simulink library "intertravamento"  (R2015a)
settings: Solver=ode45  SolverMode=SingleTasking  StartTime=0.0  StopTime=10.0  RelTol=1e-3
PostLoadFcn:
  | setsysloc_simulink(bdroot)
undefined symbols (not defined in the file or in its folder): docblock, getdatatypespecs, NumBits1, NumBits2, sfunxy, sigbuilder_block, slcm, SlDemoSign, Slope1, Slope2
libraries: simulink x46, sl_helperblocks x2, eml_lib x1
(part 6 of 6)

== system intertravamento/Model-Wide Utilities/Block Support Table ==
  EmptySubsystem : Subsystem

== system intertravamento/Model-Wide Utilities/DocBlock ==
  EmptySubsystem : Subsystem

== system intertravamento/Model-Wide Utilities/Model Info ==
  EmptySubsystem : Subsystem

== system intertravamento/Model-Wide Utilities/Timed-Based Linearization ==
  Clock : Clock
      settings: DisableCoverage=on
  Constant : Constant  DisableCoverage=on  Value=LinearizationTime
  Sum : Sum  DisableCoverage=on  Inputs=-+  SaturateOnIntegerOverflow=on  InputSameDT=on  OutDataTypeStr=Inherit: Same as first input
  Triggered Linearization : Subsystem  DisableCoverage=on  TreatAsAtomicUnit=on
  wires:
  Clock/1 -> Sum/2
  Constant/1 -> Sum/1
  Sum/1 -> Triggered Linearization/Trigger

== system intertravamento/Model-Wide Utilities/Trigger-Based Linearization ==
  Trigger : TriggerPort
  MATLAB S-Function : M-S-Function  DisableCoverage=on  FunctionName=sfunlin  Parameters=name_,SampleTime

== system intertravamento/Ports & Subsystems/Atomic Subsystem ==
  In1 : Inport
  Out1 : Outport
  wires:
  In1/1 -> Out1/1

== system intertravamento/Ports & Subsystems/CodeReuseSubsystem ==
  In1 : Inport
  Out1 : Outport
  wires:
  In1/1 -> Out1/1

== system intertravamento/Ports & Subsystems/Configurable Subsystem ==

== system intertravamento/Ports & Subsystems/Enabled Subsystem ==
  In1 : Inport
  Enable : EnablePort
  Out1 : Outport
  wires:
  In1/1 -> Out1/1

== system intertravamento/Ports & Subsystems/Enabled and Triggered Subsystem ==
  In1 : Inport
  Enable : EnablePort
  Trigger : TriggerPort
  Out1 : Outport
  wires:
  In1/1 -> Out1/1

== system intertravamento/Ports & Subsystems/For Each Subsystem ==
  In1 : Inport  Partition=on  PartitionDimension=1  PartitionWidth=1
  For Each : ForEach  DisableCoverage=on  IndexMode=One-based
  Out1 : Outport  ConcatenationDimension=1
  wires:
  In1/1 -> Out1/1

== system intertravamento/Ports & Subsystems/For Iterator Subsystem ==
  In1 : Inport
  For Iterator : ForIterator
  Out1 : Outport
  wires:
  In1/1 -> Out1/1

== system intertravamento/Ports & Subsystems/Function-Call Subsystem ==
  In1 : Inport
  function : TriggerPort  TriggerType=function-call
  Out1 : Outport
  wires:
  In1/1 -> Out1/1

== system intertravamento/Ports & Subsystems/If Action Subsystem ==
  In1 : Inport
  Action Port : ActionPort  ActionType=then
  Out1 : Outport
  wires:
  In1/1 -> Out1/1

== system intertravamento/Ports & Subsystems/Resettable Subsystem ==
  In1 : Inport
  Reset : ResetPort  DisableCoverage=on
  Out1 : Outport
  wires:
  In1/1 -> Out1/1

== system intertravamento/Ports & Subsystems/Subsystem ==
  In1 : Inport
  Out1 : Outport
  wires:
  In1/1 -> Out1/1

== system intertravamento/Ports & Subsystems/Subsystem Examples ==
  Gain : Gain  SaturateOnIntegerOverflow=on  OutDataTypeStr=Inherit: Same as input  ParamDataTypeStr=Inherit: Same as input

== system intertravamento/Ports & Subsystems/Switch Case Action Subsystem ==
  In1 : Inport
  Action Port : ActionPort  ActionType=case
  Out1 : Outport
  wires:
  In1/1 -> Out1/1

== system intertravamento/Ports & Subsystems/Triggered Subsystem ==
  In1 : Inport
  Trigger : TriggerPort
  Out1 : Outport
  wires:
  In1/1 -> Out1/1

== system intertravamento/Ports & Subsystems/Variant Subsystem ==
  note: 1) Add Subsystem or Model blocks as valid variant choices.
      | 2) You cannot connect blocks at this level. At simulation, connectivity is automatically
      | determined, based on the active variant and port name matching.
  In1 : Inport
  Out1 : Outport

== system intertravamento/Ports & Subsystems/While Iterator Subsystem ==
  In1 : Inport
  IC : Inport  Port=2
  While Iterator : WhileIterator
  Out1 : Outport
  wires:
  In1/1 -> Out1/1
  IC/1 -> While Iterator/2

== system intertravamento/Signal Attributes/Data Type Conversion Inherited ==
  DTS reference : Inport
  u : Inport  Port=2
  Conversion : DataTypeConversion  LockScale=on
  Data Type Duplicate : DataTypeDuplicate  DisableCoverage=on
  y : Outport
  wires:
  u/1 -> Conversion/1
  DTS reference/1 -> Data Type Duplicate/1
  Conversion/1 -> y/1, Data Type Duplicate/2

== system intertravamento/Signal Attributes/Data Type Propagation Examples ==
  Gain : Gain  SaturateOnIntegerOverflow=on  OutDataTypeStr=Inherit: Same as input  ParamDataTypeStr=Inherit: Same as input

== system intertravamento/Signal Attributes/Data Type Scaling Strip ==
  note: Force Scaling to be nominal,
      | slope == 1.0
      | bias == 0.0
  note: Gateway Out set to "auto"
      | which is similar to
      | "Inherit via back propagation"
  u : Inport
  FixPt Data Type Propagation : simulink/Signal Attributes/Data Type Propagation  PropDataType=fixdt(1, 16)  IfRefDouble=double  IfRefSingle=single  IsSigned=IsSigned1  NumBitsBase=NumBits1  NumBitsMult=1  NumBitsAdd=0  NumBitsAllowFinal=[8,16,32,128]  PropScalingMode=Specify via dialog  PropScaling=1  ValuesUsedBestPrec=[5 -7]  SlopeBase=Slope1  SlopeMult=0  SlopeAdd=1  BiasBase=Bias1  BiasMult=1  BiasAdd=0
  FixPt Gateway Out : DataTypeConversion  ConvertRealWorld=Stored Integer (SI)
  y : Outport
  wires:
  u/1 -> FixPt Data Type Propagation/1, FixPt Data Type Propagation/2, FixPt Gateway Out/1
  FixPt Gateway Out/1 -> FixPt Data Type Propagation/3, y/1

== system intertravamento/Signal Routing/Environment Controller ==
  Sim : Inport
  Coder : Inport  Port=2
  Environment Switch : Switch  DisableCoverage=on  Criteria=u2 ~= 0  ZeroCross=off  InputSameDT=on
  Numerical Unity : SignalConversion
  Switch Control : Constant  DisableCoverage=on  Value=switch_mode  OutDataTypeStr=boolean
  Out : Outport
  wires:
  Sim/1 -> Environment Switch/1
  Switch Control/1 -> Environment Switch/2
  Environment Switch/1 -> Numerical Unity/1
  Coder/1 -> Environment Switch/3
  Numerical Unity/1 -> Out/1

== system intertravamento/Sinks/XY Graph ==
  x : Inport
  y : Inport  Port=2
  Data Type Conversion : DataTypeConversion  DisableCoverage=on  OutDataTypeStr=double
  Data Type Conversion1 : DataTypeConversion  DisableCoverage=on  OutDataTypeStr=double
  Mux : Mux  Inputs=2
  sfunxy : S-Function  DisableCoverage=on  FunctionName=sfunxy  Parameters=[xmin xmax ymin ymax], st
  wires:
  Mux/1 -> sfunxy/1
  x/1 -> Data Type Conversion/1
  y/1 -> Data Type Conversion1/1
  Data Type Conversion/1 -> Mux/1
  Data Type Conversion1/1 -> Mux/2

== system intertravamento/Sources/Band-Limited White Noise ==
  Output : Gain  Gain=[sqrt(Cov)]/[sqrt(Ts)]  SaturateOnIntegerOverflow=on  OutDataTypeStr=Inherit: Same as input  ParamDataTypeStr=Inherit: Same as input
  White Noise : RandomNumber  DisableCoverage=on  Seed=seed  SampleTime=Ts
  y : Outport
  wires:
  White Noise/1 -> Output/1
  Output/1 -> y/1

== system intertravamento/Sources/Chirp Signal ==
  note: freqSlope = deltaFreq/targetTime;
      | instantaneousFreq(t) = freqSlope*t + initialFreq;
      | intantaneousPhase(t) = integral(instFreq) = ...
      |       0.5*freqSlope*t^2 + initialFreq*t;
      | outputSignal(t) = sin(instantaneousPhase(t));
  Clock1 : Clock
      settings: DisableCoverage=on
  Gain : Gain  DisableCoverage=on  Gain=0.5  OutDataTypeStr=Inherit: Same as input  ParamDataTypeStr=Inherit: Same as input
  Output : Trigonometry
  Product : Product  DisableCoverage=on  Inputs=*/  SaturateOnIntegerOverflow=on  InputSameDT=on  OutDataTypeStr=Inherit: Same as first input
  Product1 : Product  DisableCoverage=on  SaturateOnIntegerOverflow=on  InputSameDT=on  OutDataTypeStr=Inherit: Same as first input
  Product2 : Product  DisableCoverage=on  SaturateOnIntegerOverflow=on  InputSameDT=on  OutDataTypeStr=Inherit: Same as first input
  Sum : Sum  DisableCoverage=on  Inputs=|++  SaturateOnIntegerOverflow=on  InputSameDT=on  OutDataTypeStr=Inherit: Same as first input
  deltaFreq : Constant  DisableCoverage=on  Value=2*pi*(f2-f1)
  initialFreq : Constant  DisableCoverage=on  Value=2*pi*f1
  targetTime : Constant  DisableCoverage=on  Value=T
  y : Outport
  wires:
  deltaFreq/1 -> Product/1
  targetTime/1 -> Product/2
  Product/1 -> Gain/1
  Clock1/1 -> Product1/1, Product2/1
  Gain/1 -> Product1/2
  Product1/1 -> Sum/1
  initialFreq/1 -> Sum/2
  Sum/1 -> Product2/2
  Product2/1 -> Output/1
  Output/1 -> y/1

== system intertravamento/Sources/Counter Free-Running ==
  FixPt Data Type Propagation : simulink/Signal Attributes/Data Type Propagation  PropDataTypeMode=Specify via dialog  PropDataType=uint(NumBits)  IfRefDouble=double  IfRefSingle=single  IsSigned=IsSigned1 or IsSigned2  NumBitsBase=max([NumBits1 NumBits2])  NumBitsMult=1  NumBitsAdd=0  NumBitsAllowFinal=1:128  PropScalingMode=Specify via dialog  PropScaling=1  ValuesUsedBestPrec=[5 -7]  SlopeBase=min([Slope1 Slope2])  SlopeMult=1  SlopeAdd=0  BiasBase=Bias1  BiasMult=1  BiasAdd=0
  Force to be scalar : SignalSpecification  DisableCoverage=on  Dimensions=1
  Increment Real World : simulink/Additional Math & Discrete/Additional Math: Increment - Decrement/Increment Real World  DisableCoverage=on
  Output : UnitDelay  InitialCondition=0.0  SampleTime=tsamp
  Wrap To Zero : simulink/Discontinuities/Wrap To Zero  DisableCoverage=on  Threshold=(2^(NumBits))-1
  y : Outport
  wires:
  Force to be scalar/1 -> Increment Real World/1
  Wrap To Zero/1 -> Output/1, FixPt Data Type Propagation/1, FixPt Data Type Propagation/3, FixPt Data Type Propagation/2
  Increment Real World/1 -> Wrap To Zero/1
  Output/1 -> Force to be scalar/1, y/1

== system intertravamento/Sources/Counter Limited ==
  Data Type Propagation : simulink/Signal Attributes/Data Type Propagation  PropDataTypeMode=Specify via dialog  PropDataType=uint(nbits)  IfRefDouble=double  IfRefSingle=single  IsSigned=IsSigned1 or IsSigned2  NumBitsBase=max([NumBits1 NumBits2])  NumBitsMult=1  NumBitsAdd=0  NumBitsAllowFinal=1:128  PropScalingMode=Specify via dialog  PropScaling=1  ValuesUsedBestPrec=[5 -7]  SlopeBase=min([Slope1 Slope2])  SlopeMult=1  SlopeAdd=0  BiasBase=Bias1  BiasMult=1  BiasAdd=0
  Force to be scalar : SignalSpecification  DisableCoverage=on  Dimensions=1
  Increment Real World : simulink/Additional Math & Discrete/Additional Math: Increment - Decrement/Increment Real World  DisableCoverage=on
  Output : UnitDelay  InitialCondition=0.0  SampleTime=tsamp
  Wrap To Zero : simulink/Discontinuities/Wrap To Zero  DisableCoverage=on  Threshold=uplimit
  y : Outport
  wires:
  Force to be scalar/1 -> Increment Real World/1
  Increment Real World/1 -> Wrap To Zero/1
  Output/1 -> Force to be scalar/1, y/1
  Wrap To Zero/1 -> Data Type Propagation/3, Data Type Propagation/2, Data Type Propagation/1, Output/1

== system intertravamento/Sources/Enumerated Constant ==
  Constant : Constant  DialogController=Simulink.DDGSource  Value=SlDemoSign.Positive  OutDataTypeStr=Enum: SlDemoSign  LockScale=on
  Out : Outport
  wires:
  Constant/1 -> Out/1

== system intertravamento/Sources/Ramp ==
  Clock : Clock
      settings: DisableCoverage=on
  Constant : Constant  DisableCoverage=on  Value=start  OutDataTypeStr=Inherit: Inherit via back propagation
  Constant1 : Constant  DisableCoverage=on  Value=X0  OutDataTypeStr=Inherit: Inherit via back propagation
  Output : Sum  Inputs=|++  SaturateOnIntegerOverflow=on  InputSameDT=on  OutDataTypeStr=Inherit: Same as first input
  Product : Product  DisableCoverage=on  SaturateOnIntegerOverflow=on  InputSameDT=on  OutDataTypeStr=Inherit: Same as first input
  Step : Step  DisableCoverage=on  Time=start  After=slope  SampleTime=0
  Sum : Sum  DisableCoverage=on  Inputs=|+-  SaturateOnIntegerOverflow=on  InputSameDT=on  OutDataTypeStr=Inherit: Same as first input
  Out1 : Outport
  wires:
  Step/1 -> Product/1
  Product/1 -> Output/1
  Constant1/1 -> Output/2
  Output/1 -> Out1/1
  Sum/1 -> Product/2
  Constant/1 -> Sum/2
  Clock/1 -> Sum/1

== system intertravamento/Sources/Repeating Sequence ==
  Clock : Clock
      settings: DisableCoverage=on
  Constant : Constant  DisableCoverage=on  Value=period
  Look-Up Table1 : Lookup_n-D  DisableCoverage=on  NumberOfTableDimensions=1  BreakpointsForDimension1=rep_seq_t - min(rep_seq_t)  BreakpointsForDimension3=[5, 7]  Table=rep_seq_y  InternalRulePriority=Speed  SaturateOnIntegerOverflow=on  InputSameDT=on
  Math Function : Math  DisableCoverage=on  Operator=rem  SaturateOnIntegerOverflow=on
  Output : SignalConversion
  Sum : Sum  DisableCoverage=on  Inputs=+-  SaturateOnIntegerOverflow=on  InputSameDT=on  OutDataTypeStr=Inherit: Same as first input
  startTime : S-Function  DisableCoverage=on  FunctionName=sfun_tstart
  Out1 : Outport
  wires:
  Math Function/1 -> Look-Up Table1/1
  Sum/1 -> Math Function/1
  Clock/1 -> Sum/1
  startTime/1 -> Sum/2
  Look-Up Table1/1 -> Output/1
  Output/1 -> Out1/1
  Constant/1 -> Math Function/2

== system intertravamento/Sources/Repeating Sequence Interpolated ==
  Data Type Propagation : simulink/Signal Attributes/Data Type Propagation  PropDataType=fixdt(1, 16)  IfRefDouble=double  IfRefSingle=single  IsSigned=IsSigned2  NumBitsBase=NumBits2  NumBitsMult=1  NumBitsAdd=0  NumBitsAllowFinal=1:128  PropScaling=2^-10  ValuesUsedBestPrec=[5 -7]  SlopeBase=Slope2  SlopeMult=1  SlopeAdd=0  BiasBase=Bias2  BiasMult=1  BiasAdd=0
  Data Type Conversion : DataTypeConversion  DisableCoverage=on
  Force to be scalar : SignalSpecification  DisableCoverage=on  Dimensions=1
  LimitedCounter : simulink/Sources/Counter Limited  uplimit=nn  tsamp=tsamp
  Lookup : Lookup_n-D  DisableCoverage=on  NumberOfTableDimensions=1  BreakpointsForDimension1=TimeValues  BreakpointsForDimension3=[5, 7]  Table=OutValues  ExtrapMethod=Clip  OutMin=OutMin  OutMax=OutMax  OutDataTypeStr=OutDataTypeStr  InputSameDT=on
  Output : SignalConversion
  Sample Time Math : SampleTimeMath  DisableCoverage=on  TsampMathOp=*  TsampMathImp=Offline Scaling Adjustment
  y : Outport  OutMin=OutMin  OutMax=OutMax
  wires:
  Output/1 -> y/1
  Lookup/1 -> Output/1, Data Type Propagation/1
  Force to be scalar/1 -> Data Type Conversion/1, Data Type Propagation/2
  LimitedCounter/1 -> Force to be scalar/1
  Sample Time Math/1 -> Lookup/1
  Data Type Conversion/1 -> Sample Time Math/1, Data Type Propagation/3

== system intertravamento/Sources/Repeating Sequence Stair ==
  Force to be scalar : SignalSpecification  DisableCoverage=on  Dimensions=1
  LimitedCounter : simulink/Sources/Counter Limited  uplimit=nn  tsamp=tsamp
  Out : SignalConversion
  Output : MultiPortSwitch  DisableCoverage=on  DataPortOrder=Zero-based contiguous  Inputs=1  zeroidx=on  OutMin=OutMin  OutMax=OutMax  SampleTime=tsamp
  Vector : Constant  DisableCoverage=on  Value=OutValues  OutMin=OutMin  OutMax=OutMax  OutDataTypeStr=OutDataTypeStr
  y : Outport  OutMin=OutMin  OutMax=OutMax
  wires:
  Force to be scalar/1 -> Output/1
  Vector/1 -> Output/2
  LimitedCounter/1 -> Force to be scalar/1
  Output/1 -> Out/1
  Out/1 -> y/1

== system intertravamento/Sources/Signal Builder ==
  Demux : Demux  Tag=STV Demux  Outputs=1
  FromWs : FromWorkspace  Tag=STV FromWs  VariableName=tuvar  SampleTime=0
      SigBuilderData=|
      | common.afterFinalStr = 'Extrapolate'
      | common.sampleTime = 0
      | dataSet.timeRange = [0 10]
      | dataSet.name = 'Group 1'
      | sbobj.Groups.Name = 'Group 1'
      | sbobj.Groups.Signals.Name = 'Signal 1'
      | sbobj.Groups.Signals.XData = [0 4 4 6 6 10]
      | sbobj.Groups.Signals.YData = [0 0 1 1 0 0]
  Signal 1 : Outport  Tag=STV Outport
  wires:
  FromWs/1 -> Demux/1
  Demux/1 -> Signal 1/1

== system intertravamento/User-Defined Functions/S-Function Examples ==
  Gain : Gain  SaturateOnIntegerOverflow=on  OutDataTypeStr=Inherit: Same as input  ParamDataTypeStr=Inherit: Same as input

== system intertravamento/User-Defined Functions/Simulink Function ==
  f : TriggerPort  TriggerType=function-call  IsSimulinkFunction=on  FunctionName=f
  u : ArgIn  DisableCoverage=on  ArgumentName=u
  y : ArgOut  DisableCoverage=on  ArgumentName=y
  wires:
  u/1 -> y/1

== system intertravamento/Additional Math & Discrete/Additional Discrete/Fixed-Point State-Space ==
  note: U(k)
  note: U(k)
  note: Y(k)
  u : Inport
  Data Type Duplicate : DataTypeDuplicate  DisableCoverage=on  NumInputPorts=3
  Data Type Duplicate1 : DataTypeDuplicate  DisableCoverage=on  NumInputPorts=3
  DataTypeProp : simulink/Signal Attributes/Data Type Propagation  PropDataType=fixdt(1, 16)  IfRefDouble=double  IfRefSingle=single  IsSigned=IsSigned1 or IsSigned2  NumBitsBase=NumBits1  NumBitsMult=1  NumBitsAdd=0  NumBitsAllowFinal=1:128  PropScaling=2^-10  ValuesUsedBestPrec=[5 -7]  SlopeBase=PosRange2  SlopeMult=1  SlopeAdd=0  BiasBase=Bias2  BiasMult=1  BiasAdd=0
  DataTypeProp1 : simulink/Signal Attributes/Data Type Propagation  PropDataType=fixdt(1, 16)  IfRefDouble=double  IfRefSingle=single  IsSigned=IsSigned1 or IsSigned2  NumBitsBase=NumBits1  NumBitsMult=1  NumBitsAdd=0  NumBitsAllowFinal=1:128  PropScaling=2^-10  ValuesUsedBestPrec=[5 -7]  SlopeBase=PosRange2  SlopeMult=1  SlopeAdd=0  BiasBase=Bias2  BiasMult=1  BiasAdd=0
  Delay State X : UnitDelay  Description=Store in Global RAM  DisableCoverage=on  InitialCondition=X0  SampleTime=-1
      settings: AttributesFormatString=%<Description>
  Direct Link Matrix D : Gain  Description=Multiply in CPU  DisableCoverage=on  Gain=D  Multiplication=Matrix(K*u) (u vector)  OutDataTypeStr=Inherit: Inherit via back propagation
      settings: AttributesFormatString=%<Description>
  Downcast Next State X : DataTypeConversion  Description=|  DisableCoverage=on
      | Reduce from CPU Size
      |  to Global RAM Size
      settings: AttributesFormatString=%<Description>
  Downcast Output Y : DataTypeConversion  Description=|
      | Reduce from CPU Size
      |  to Global RAM Size
      settings: AttributesFormatString=%<Description>
  Input Matrix B : Gain  Description=Multiply in CPU  DisableCoverage=on  Gain=B  Multiplication=Matrix(K*u) (u vector)  OutDataTypeStr=Inherit: Inherit via back propagation
      settings: AttributesFormatString=%<Description>
  Output Matrix C : Gain  Description=Multiply in CPU  DisableCoverage=on  Gain=C  Multiplication=Matrix(K*u) (u vector)  OutDataTypeStr=Inherit: Inherit via back propagation
      settings: AttributesFormatString=%<Description>
  State Matrix A : Gain  Description=Multiply in CPU  DisableCoverage=on  Gain=A  Multiplication=Matrix(K*u) (u vector)  OutDataTypeStr=Inherit: Inherit via back propagation
      settings: AttributesFormatString=%<Description>
  Sum Output Equation : Sum  Description=Add in CPU  DisableCoverage=on  OutDataTypeStr=slDataTypeAndScale(('InternalDataType'),('OutputEqScaling'))
      settings: AttributesFormatString=%<Description>
  Sum State Equation : Sum  Description=Add in CPU  DisableCoverage=on  OutDataTypeStr=slDataTypeAndScale(('InternalDataType'),('StateEqScaling'))
      settings: AttributesFormatString=%<Description>
  y : Outport  InitialOutput=0
  wires:
  Direct Link Matrix D/1 -> Data Type Duplicate1/3, Sum Output Equation/1  "DU(k)"
  Output Matrix C/1 -> Data Type Duplicate1/2, Sum Output Equation/2  "CX(k)"
  Sum Output Equation/1 -> DataTypeProp/2, Data Type Duplicate1/1, Downcast Output Y/1  "CX(k)+DU(k)"
  Downcast Output Y/1 -> DataTypeProp/3, y/1
  Delay State X/1 -> Output Matrix C/1, State Matrix A/1  "X(k)"
  Downcast Next State X/1 -> DataTypeProp1/3, Delay State X/1  "X(k+1)"
  Sum State Equation/1 -> DataTypeProp1/2, Data Type Duplicate/1, Downcast Next State X/1  "AX(k)+BU(k)"
  Input Matrix B/1 -> Data Type Duplicate/3, Sum State Equation/1  "BU(k)"
  u/1 -> DataTypeProp1/1, DataTypeProp/1, Direct Link Matrix D/1, Input Matrix B/1
  State Matrix A/1 -> Data Type Duplicate/2, Sum State Equation/2  "AX(k)"

== system intertravamento/Additional Math & Discrete/Additional Discrete/Transfer Fcn Direct Form II ==
  u : Inport
  DataTypeProp : simulink/Signal Attributes/Data Type Propagation  PropDataType=fixdt(1, 16)  IfRefDouble=double  IfRefSingle=single  IsSigned=IsSigned1 or IsSigned2  NumBitsBase=max([NumBits1 NumBits2])  NumBitsMult=1  NumBitsAdd=0  NumBitsAllowFinal=1:128  PropScaling=2^-10  ValuesUsedBestPrec=[5 -7]  SlopeBase=min([Slope1 Slope2])  SlopeMult=OutputSlopeMult  SlopeAdd=0  BiasBase=Bias1  BiasMult=0  BiasAdd=0
  DataTypeProp1 : simulink/Signal Attributes/Data Type Propagation  PropDataType=fixdt(1, 16)  IfRefDouble=double  IfRefSingle=single  IsSigned=IsSigned1 or IsSigned2  NumBitsBase=max([NumBits1 NumBits2])  NumBitsMult=1  NumBitsAdd=0  NumBitsAllowFinal=1:128  PropScaling=2^-10  ValuesUsedBestPrec=[5 -7]  SlopeBase=min([Slope1 Slope2])  SlopeMult=OutputSlopeMult2  SlopeAdd=0  BiasBase=Bias1  BiasMult=0  BiasAdd=0
  DenCoef : Gain  DisableCoverage=on  Gain=DenCoefVec  Multiplication=Matrix(K*u) (u vector)
      settings: AttributesFormatString=|
      | Data Type and Scaling Inherited
      | with goal of NO Quantization Noise
      | Possible Overflow or Saturation
  Downcast : DataTypeConversion  Description=|  LockScale=on
      | Reduce from CPU Size
      |  to Global RAM Size
      settings: AttributesFormatString=%<Description>
  Downcast1 : DataTypeConversion  Description=|  DisableCoverage=on  LockScale=on
      | Reduce from CPU Size
      |  to Global RAM Size
      settings: AttributesFormatString=%<Description>
  Mux : Mux  Inputs=2
  NumCoef : Gain  DisableCoverage=on  Gain=NumCoefVec  Multiplication=Matrix(K*u) (u vector)
      settings: AttributesFormatString=|
      | Data Type and Scaling Inherited
      | with goal of NO Quantization Noise
      | Possible Overflow or Saturation
  Sum : Sum  Tag=S16 2^-10  DisableCoverage=on  Inputs=+-  LockScale=on
      settings: AttributesFormatString=|
      | Data Type and Scaling Inherited
      | with goal of NO Quantization Noise
      | Possible Overflow or Saturation
  Tapped Delay : simulink/Discrete/Tapped Delay  vinit=vinit  samptime=-1  NumDelays=-1  DelayOrder=Newest  includeCurrent=off
      settings: AttributesFormatString=|
      | Number of Taps
      | Inherited via Back Propagation
  y : Outport
  wires:
  Sum/1 -> Downcast1/1
  DenCoef/1 -> Sum/2
  u/1 -> DataTypeProp1/1, DataTypeProp1/2, DataTypeProp/2, DataTypeProp/1, Sum/1
  NumCoef/1 -> Downcast/1
  Tapped Delay/1 -> DenCoef/1, Mux/2
  Downcast1/1 -> DataTypeProp1/3, Mux/1, Tapped Delay/1
  Mux/1 -> NumCoef/1
  Downcast/1 -> y/1, DataTypeProp/3

== system intertravamento/Additional Math & Discrete/Additional Discrete/Transfer Fcn Direct Form II Time Varying ==
  u : Inport
  Num : Inport  Port=2
  Den No Lead : Inport  Port=3
  DataTypeProp : simulink/Signal Attributes/Data Type Propagation  PropDataType=fixdt(1, 16)  IfRefDouble=double  IfRefSingle=single  IsSigned=IsSigned1  NumBitsBase=NumBits1  NumBitsMult=1  NumBitsAdd=0  NumBitsAllowFinal=1:128  PropScaling=2^-10  ValuesUsedBestPrec=[5 -7]  SlopeBase=Slope1  SlopeMult=1  SlopeAdd=0  BiasBase=Bias1  BiasMult=1  BiasAdd=0
  DataTypeProp1 : simulink/Signal Attributes/Data Type Propagation  PropDataType=fixdt(1, 16)  IfRefDouble=double  IfRefSingle=single  IsSigned=IsSigned1  NumBitsBase=NumBits1  NumBitsMult=1  NumBitsAdd=0  NumBitsAllowFinal=1:128  PropScaling=2^-10  ValuesUsedBestPrec=[5 -7]  SlopeBase=Slope1  SlopeMult=2  SlopeAdd=0  BiasBase=Bias1  BiasMult=1  BiasAdd=0
  Dot1 : DotProduct  DisableCoverage=on  OutDataTypeStr=Inherit: Inherit via internal rule
      settings: AttributesFormatString=|
      | Data Type and Scaling Inherited
      | with goal of NO Quantization Noise
      | Possible Overflow or Saturation
  Dot2 : DotProduct  DisableCoverage=on  OutDataTypeStr=Inherit: Inherit via internal rule
      settings: AttributesFormatString=|
      | Data Type and Scaling Inherited
      | with goal of NO Quantization Noise
      | Possible Overflow or Saturation
  Downcast : DataTypeConversion  Description=|  LockScale=on
      | Reduce from CPU Size
      |  to Global RAM Size
      settings: AttributesFormatString=%<Description>
  Downcast1 : DataTypeConversion  Description=|  DisableCoverage=on  LockScale=on
      | Reduce from CPU Size
      |  to Global RAM Size
      settings: AttributesFormatString=%<Description>
  Mux : Mux  Inputs=2
  Sum : Sum  Tag=S16 2^-10  DisableCoverage=on  Inputs=+-  LockScale=on
      settings: AttributesFormatString=|
      | Data Type and Scaling Inherited
      | with goal of NO Quantization Noise
      | Possible Overflow or Saturation
  Tapped Delay : simulink/Discrete/Tapped Delay  vinit=vinit  samptime=-1  NumDelays=-1  DelayOrder=Newest  includeCurrent=off
      settings: AttributesFormatString=|
      | Number of Taps
      | Inherited via Back Propagation
  y : Outport
  wires:
  Den No Lead/1 -> Dot1/2
  Num/1 -> Dot2/2
  Downcast/1 -> DataTypeProp/3, y/1
  Mux/1 -> Dot2/1
  Downcast1/1 -> DataTypeProp1/3, Tapped Delay/1, Mux/1
  Tapped Delay/1 -> Dot1/1, Mux/2
  Dot2/1 -> Downcast/1
  u/1 -> Sum/1, DataTypeProp1/2, DataTypeProp1/1, DataTypeProp/2, DataTypeProp/1
  Dot1/1 -> Sum/2
  Sum/1 -> Downcast1/1

== system intertravamento/Additional Math & Discrete/Additional Discrete/Unit Delay Enabled ==
  note: Enable
  note: Xold
  u : Inport
  E : Inport  Port=2
  Enable : Switch  Criteria=u2 ~= 0  OutDataTypeStr=Inherit: Inherit via back propagation  ZeroCross=off
  FixPt Data Type Duplicate1 : DataTypeDuplicate  DisableCoverage=on  NumInputPorts=3
  FixPt Unit Delay1 : UnitDelay  InitialCondition=vinit  SampleTime=tsamp  HasFrameUpgradeWarning=off
  y : Outport
  wires:
  E/1 -> Enable/2
  u/1 -> FixPt Data Type Duplicate1/3, Enable/1
  Enable/1 -> FixPt Unit Delay1/1, FixPt Data Type Duplicate1/2  "Xnew"
  FixPt Unit Delay1/1 -> y/1, Enable/3, FixPt Data Type Duplicate1/1

== system intertravamento/Additional Math & Discrete/Additional Discrete/Unit Delay Enabled External IC ==
  note: Enable
  note: Initial Value
  u : Inport
  E : Inport  Port=2
  IC : Inport  Port=3
  Enable : Switch  Criteria=u2 ~= 0  OutDataTypeStr=Inherit: Inherit via back propagation  ZeroCross=off
  FixPt Data Type Duplicate1 : DataTypeDuplicate  DisableCoverage=on  NumInputPorts=4
  Unit Delay External IC : simulink/Additional Math & Discrete/Additional Discrete/Unit Delay External IC  tsamp=tsamp
  y : Outport
  wires:
  E/1 -> Enable/2
  IC/1 -> FixPt Data Type Duplicate1/3, Unit Delay External IC/2
  u/1 -> FixPt Data Type Duplicate1/4, Enable/1
  Enable/1 -> FixPt Data Type Duplicate1/2, Unit Delay External IC/1  "Xnew"
  Unit Delay External IC/1 -> y/1, Enable/3, FixPt Data Type Duplicate1/1

== system intertravamento/Additional Math & Discrete/Additional Discrete/Unit Delay Enabled Resettable ==
  note: Enable
  note: Reset
  u : Inport
  E : Inport  Port=2
  R : Inport  Port=3
  Enable : Switch  Criteria=u2 ~= 0  OutDataTypeStr=Inherit: Inherit via back propagation  ZeroCross=off
  FixPt Data Type Duplicate2 : DataTypeDuplicate  DisableCoverage=on  NumInputPorts=3
  Unit Delay Resettable : simulink/Additional Math & Discrete/Additional Discrete/Unit Delay Resettable  vinit=vinit  tsamp=tsamp
  y : Outport
  wires:
  E/1 -> Enable/2
  u/1 -> Enable/1, FixPt Data Type Duplicate2/3
  Enable/1 -> FixPt Data Type Duplicate2/2, Unit Delay Resettable/1  "Xnew"
  Unit Delay Resettable/1 -> FixPt Data Type Duplicate2/1, Enable/3, y/1
  R/1 -> Unit Delay Resettable/2

== system intertravamento/Additional Math & Discrete/Additional Discrete/Unit Delay Enabled Resettable External IC ==
  note: Enable
  note: Reset
  note: Initial Value
  u : Inport
  E : Inport  Port=2
  R : Inport  Port=3
  IC : Inport  Port=4
  Enable : Switch  Criteria=u2 ~= 0  OutDataTypeStr=Inherit: Inherit via back propagation  ZeroCross=off
  FixPt Data Type Duplicate1 : DataTypeDuplicate  DisableCoverage=on  NumInputPorts=4
  Unit Delay Resettable External IC : simulink/Additional Math & Discrete/Additional Discrete/Unit Delay Resettable External IC  tsamp=tsamp
  y : Outport
  wires:
  Unit Delay Resettable External IC/1 -> y/1, Enable/3, FixPt Data Type Duplicate1/1
  R/1 -> Unit Delay Resettable External IC/2
  Enable/1 -> Unit Delay Resettable External IC/1, FixPt Data Type Duplicate1/3
  u/1 -> Enable/1, FixPt Data Type Duplicate1/4
  IC/1 -> Unit Delay Resettable External IC/3, FixPt Data Type Duplicate1/2
  E/1 -> Enable/2

== system intertravamento/Additional Math & Discrete/Additional Discrete/Unit Delay External IC ==
  note: Xnew
  note: Initial Value
  u : Inport
  IC : Inport  Port=2
  FixPt Constant : Constant  DisableCoverage=on  Value=0  OutDataTypeStr=fixdt(0,8,0)
  FixPt Data Type Duplicate1 : DataTypeDuplicate  DisableCoverage=on  NumInputPorts=3
  FixPt Unit Delay1 : UnitDelay  DisableCoverage=on  InitialCondition=0.0  SampleTime=tsamp  HasFrameUpgradeWarning=off
  FixPt Unit Delay2 : UnitDelay  DisableCoverage=on  InitialCondition=1  SampleTime=tsamp
  Init : Switch  Criteria=u2 ~= 0  OutDataTypeStr=Inherit: Inherit via back propagation  ZeroCross=off
  y : Outport
  wires:
  FixPt Unit Delay1/1 -> Init/3  "Xold"
  Init/1 -> y/1, FixPt Data Type Duplicate1/1
  FixPt Unit Delay2/1 -> Init/2
  FixPt Constant/1 -> FixPt Unit Delay2/1
  u/1 -> FixPt Unit Delay1/1, FixPt Data Type Duplicate1/2
  IC/1 -> Init/1, FixPt Data Type Duplicate1/3

== system intertravamento/Additional Math & Discrete/Additional Discrete/Unit Delay Resettable ==
  note: Reset
  u : Inport
  R : Inport  Port=2
  FixPt Constant : Constant  DisableCoverage=on  Value=0  OutDataTypeStr=fixdt(0,8,0)
  FixPt Data Type Duplicate1 : DataTypeDuplicate  DisableCoverage=on  NumInputPorts=4
  FixPt Logical Operator : Logic  DisableCoverage=on  Operator=OR  AllPortsSameDT=off  OutDataTypeStr=fixdt(0, 8)
  FixPt Unit Delay1 : UnitDelay  DisableCoverage=on  InitialCondition=vinit  SampleTime=tsamp  HasFrameUpgradeWarning=off
  FixPt Unit Delay2 : UnitDelay  DisableCoverage=on  InitialCondition=1  SampleTime=tsamp
  Init : Switch  Criteria=u2 ~= 0  OutDataTypeStr=Inherit: Inherit via back propagation  ZeroCross=off
  Initial Condition : Constant  DisableCoverage=on  Value=vinit  OutDataTypeStr=Inherit: Inherit via back propagation
  Reset : Switch  Criteria=u2 ~= 0  OutDataTypeStr=Inherit: Inherit via back propagation  ZeroCross=off
  y : Outport
  wires:
  Initial Condition/1 -> Reset/1, Init/1, FixPt Data Type Duplicate1/3  "Initial Value"
  u/1 -> FixPt Data Type Duplicate1/4, Reset/3
  Reset/1 -> FixPt Data Type Duplicate1/2, FixPt Unit Delay1/1  "Xnew"
  R/1 -> Reset/2, FixPt Logical Operator/1
  FixPt Constant/1 -> FixPt Unit Delay2/1
  FixPt Unit Delay2/1 -> FixPt Logical Operator/2
  Init/1 -> FixPt Data Type Duplicate1/1, y/1
  FixPt Unit Delay1/1 -> Init/3  "Xold"
  FixPt Logical Operator/1 -> Init/2

== system intertravamento/Additional Math & Discrete/Additional Discrete/Unit Delay Resettable External IC ==
  note: Initial Value
  note: Reset
  u : Inport
  R : Inport  Port=2
  IC : Inport  Port=3
  FixPt Constant : Constant  DisableCoverage=on  Value=0  OutDataTypeStr=fixdt(0,8,0)
  FixPt Data Type Duplicate1 : DataTypeDuplicate  DisableCoverage=on  NumInputPorts=4
  FixPt Logical Operator : Logic  DisableCoverage=on  Operator=OR  AllPortsSameDT=off  OutDataTypeStr=fixdt(0, 8)
  FixPt Unit Delay1 : UnitDelay  DisableCoverage=on  InitialCondition=0.0  SampleTime=tsamp  HasFrameUpgradeWarning=off
  FixPt Unit Delay2 : UnitDelay  DisableCoverage=on  InitialCondition=1  SampleTime=tsamp
  Init : Switch  Criteria=u2 ~= 0  OutDataTypeStr=Inherit: Inherit via back propagation  ZeroCross=off
  Reset : Switch  Criteria=u2 ~= 0  OutDataTypeStr=Inherit: Inherit via back propagation  ZeroCross=off
  y : Outport
  wires:
  IC/1 -> Reset/1, Init/1, FixPt Data Type Duplicate1/3
  u/1 -> FixPt Data Type Duplicate1/4, Reset/3
  Reset/1 -> FixPt Data Type Duplicate1/2, FixPt Unit Delay1/1  "Xnew"
  R/1 -> Reset/2, FixPt Logical Operator/1
  FixPt Constant/1 -> FixPt Unit Delay2/1
  FixPt Unit Delay2/1 -> FixPt Logical Operator/2
  Init/1 -> FixPt Data Type Duplicate1/1, y/1
  FixPt Unit Delay1/1 -> Init/3  "Xold"
  FixPt Logical Operator/1 -> Init/2

== system intertravamento/Additional Math & Discrete/Additional Discrete/Unit Delay With Preview Enabled ==
  note: Enable
  note: Xnew
  note: Xnew
  note: Xold
  u : Inport
  E : Inport  Port=2
  Enable : Switch  Criteria=u2 ~= 0  OutDataTypeStr=Inherit: Inherit via back propagation  ZeroCross=off
  FixPt Data Type Duplicate1 : DataTypeDuplicate  DisableCoverage=on  NumInputPorts=3
  FixPt Unit Delay1 : UnitDelay  InitialCondition=vinit  SampleTime=tsamp  HasFrameUpgradeWarning=off
  y : Outport
  x : Outport  Port=2
  wires:
  FixPt Unit Delay1/1 -> FixPt Data Type Duplicate1/1, Enable/3, x/1
  Enable/1 -> FixPt Data Type Duplicate1/2, FixPt Unit Delay1/1, y/1
  u/1 -> Enable/1, FixPt Data Type Duplicate1/3
  E/1 -> Enable/2

== system intertravamento/Additional Math & Discrete/Additional Discrete/Unit Delay With Preview Enabled Resettable ==
  note: Enable
  note: Xold
  note: Xnew
  note: Reset
  u : Inport
  E : Inport  Port=2
  R : Inport  Port=3
  Enable : Switch  Criteria=u2 ~= 0  OutDataTypeStr=Inherit: Inherit via back propagation  ZeroCross=off
  FixPt Data Type Duplicate2 : DataTypeDuplicate  DisableCoverage=on  NumInputPorts=5
  FixPt Unit Delay1 : UnitDelay  InitialCondition=vinit  SampleTime=tsamp  HasFrameUpgradeWarning=off
  Initial Condition : Constant  DisableCoverage=on  Value=vinit  OutDataTypeStr=Inherit: Inherit via back propagation
  Reset : Switch  Criteria=u2 ~= 0  OutDataTypeStr=Inherit: Inherit via back propagation  InputSameDT=on
  y : Outport
  x : Outport  Port=2
  wires:
  E/1 -> Enable/2
  Initial Condition/1 -> FixPt Data Type Duplicate2/3, Reset/1  "Reset Value"
  u/1 -> FixPt Data Type Duplicate2/5, Enable/1
  Enable/1 -> FixPt Data Type Duplicate2/4, Reset/3
  FixPt Unit Delay1/1 -> x/1, Enable/3, FixPt Data Type Duplicate2/1
  Reset/1 -> y/1, FixPt Data Type Duplicate2/2, FixPt Unit Delay1/1
  R/1 -> Reset/2

== system intertravamento/Additional Math & Discrete/Additional Discrete/Unit Delay With Preview Enabled Resettable External RV ==
  note: Enable
  note: Input
  note: Reset
  note: Reset Value
  note: Xnew
  note: Xold
  u : Inport
  E : Inport  Port=2
  R : Inport  Port=3
  V : Inport  Port=4
  Enable : Switch  Criteria=u2 ~= 0  OutDataTypeStr=Inherit: Inherit via back propagation  ZeroCross=off
  FixPt Data Type Duplicate2 : DataTypeDuplicate  DisableCoverage=on  NumInputPorts=5
  FixPt Unit Delay1 : UnitDelay  InitialCondition=vinit  SampleTime=tsamp  HasFrameUpgradeWarning=off
  Reset : Switch  Criteria=u2 ~= 0  OutDataTypeStr=Inherit: Inherit via back propagation  InputSameDT=on
  y1 : Outport
  y2 : Outport  Port=2
  wires:
  R/1 -> Reset/2
  Reset/1 -> FixPt Unit Delay1/1, FixPt Data Type Duplicate2/2, y1/1
  FixPt Unit Delay1/1 -> FixPt Data Type Duplicate2/1, Enable/3, y2/1
  Enable/1 -> Reset/3, FixPt Data Type Duplicate2/4
  u/1 -> Enable/1, FixPt Data Type Duplicate2/5
  V/1 -> Reset/1, FixPt Data Type Duplicate2/3
  E/1 -> Enable/2

== system intertravamento/Additional Math & Discrete/Additional Discrete/Unit Delay With Preview Resettable ==
  note: Reset
  note: Xnew
  note: Xold
  u : Inport
  R : Inport  Port=2
  FixPt Data Type Duplicate2 : DataTypeDuplicate  DisableCoverage=on  NumInputPorts=4
  FixPt Unit Delay1 : UnitDelay  InitialCondition=vinit  SampleTime=tsamp  HasFrameUpgradeWarning=off
  Initial Condition : Constant  DisableCoverage=on  Value=vinit  OutDataTypeStr=Inherit: Inherit via back propagation
  Reset : Switch  Criteria=u2 ~= 0  OutDataTypeStr=Inherit: Inherit via back propagation  ZeroCross=off
  y : Outport
  x : Outport  Port=2
  wires:
  Initial Condition/1 -> FixPt Data Type Duplicate2/3, Reset/1  "Reset Value"
  u/1 -> Reset/3, FixPt Data Type Duplicate2/4
  FixPt Unit Delay1/1 -> x/1, FixPt Data Type Duplicate2/1
  Reset/1 -> y/1, FixPt Data Type Duplicate2/2, FixPt Unit Delay1/1
  R/1 -> Reset/2

== system intertravamento/Additional Math & Discrete/Additional Discrete/Unit Delay With Preview Resettable External RV ==
  note: Reset Value
  note: Reset
  note: Xnew
  note: Xold
  u : Inport
  R : Inport  Port=2
  RV : Inport  Port=3
  FixPt Data Type Duplicate2 : DataTypeDuplicate  DisableCoverage=on  NumInputPorts=4
  FixPt Unit Delay1 : UnitDelay  InitialCondition=vinit  SampleTime=tsamp  HasFrameUpgradeWarning=off
  Reset : Switch  Criteria=u2 ~= 0  OutDataTypeStr=Inherit: Inherit via back propagation  ZeroCross=off
  y : Outport
  x : Outport  Port=2
  wires:
  RV/1 -> FixPt Data Type Duplicate2/3, Reset/1
  FixPt Unit Delay1/1 -> x/1, FixPt Data Type Duplicate2/1
  Reset/1 -> y/1, FixPt Data Type Duplicate2/2, FixPt Unit Delay1/1
  R/1 -> Reset/2
  u/1 -> Reset/3, FixPt Data Type Duplicate2/4

== system intertravamento/Additional Math & Discrete/Additional Math: Increment - Decrement/Decrement Real World ==
  u : Inport
  FixPt Constant : Constant  DisableCoverage=on  OutDataTypeStr=Inherit: Inherit via back propagation
  FixPt Data Type Duplicate : DataTypeDuplicate  DisableCoverage=on  NumInputPorts=3
  FixPt Sum1 : Sum  Inputs=+-  OutDataTypeStr=Inherit: Inherit via back propagation  InputSameDT=on  LockScale=on
  y : Outport
  wires:
  FixPt Sum1/1 -> y/1, FixPt Data Type Duplicate/1
  FixPt Constant/1 -> FixPt Sum1/2, FixPt Data Type Duplicate/3
  u/1 -> FixPt Sum1/1, FixPt Data Type Duplicate/2

== system intertravamento/Additional Math & Discrete/Additional Math: Increment - Decrement/Decrement Stored Integer ==
  u : Inport
  FixPt Constant : Constant  DisableCoverage=on  OutDataTypeStr=Inherit: Inherit via back propagation
  FixPt Data Type Duplicate : DataTypeDuplicate  DisableCoverage=on  NumInputPorts=3
  FixPt Data Type Propagation : simulink/Signal Attributes/Data Type Propagation  PropDataType=fixdt(1, 16)  IfRefDouble=double  IfRefSingle=single  IsSigned=IsSigned1  NumBitsBase=NumBits1  NumBitsMult=1  NumBitsAdd=0  NumBitsAllowFinal=1:128  PropScaling=2^-10  ValuesUsedBestPrec=[5 -7]  SlopeBase=Slope1  SlopeMult=0  SlopeAdd=1  BiasBase=Bias1  BiasMult=0  BiasAdd=0
  FixPt Gateway In : DataTypeConversion  DisableCoverage=on  ConvertRealWorld=Stored Integer (SI)
  FixPt Sum1 : Sum  Inputs=+-  OutDataTypeStr=Inherit: Inherit via back propagation  InputSameDT=on  LockScale=on
  y : Outport
  wires:
  u/1 -> FixPt Data Type Duplicate/2, FixPt Sum1/1
  FixPt Constant/1 -> FixPt Gateway In/1, FixPt Data Type Propagation/3
  FixPt Sum1/1 -> FixPt Data Type Duplicate/1, y/1
  FixPt Gateway In/1 -> FixPt Data Type Duplicate/3, FixPt Sum1/2, FixPt Data Type Propagation/1, FixPt Data Type Propagation/2

== system intertravamento/Additional Math & Discrete/Additional Math: Increment - Decrement/Decrement To Zero ==
  u : Inport
  FixPt Constant : Constant  DisableCoverage=on  OutDataTypeStr=Inherit: Inherit via back propagation
  FixPt Data Type Duplicate : DataTypeDuplicate  DisableCoverage=on  NumInputPorts=5
  FixPt Relational Operator3 : RelationalOperator  DisableCoverage=on  Operator=>  OutDataTypeStr=boolean  ZeroCross=off
  FixPt Sum1 : Sum  DisableCoverage=on  Inputs=+-  OutDataTypeStr=Inherit: Inherit via back propagation  LockScale=on
  FixPt Switch4 : Switch  Criteria=u2 ~= 0  Threshold=1  OutDataTypeStr=Inherit: Inherit via back propagation  ZeroCross=off
  Ground1 : Ground  DisableCoverage=on
  y : Outport
  wires:
  FixPt Switch4/1 -> FixPt Data Type Duplicate/1, y/1
  Ground1/1 -> FixPt Data Type Duplicate/2, FixPt Switch4/3
  FixPt Relational Operator3/1 -> FixPt Switch4/2
  u/1 -> FixPt Relational Operator3/1, FixPt Data Type Duplicate/4, FixPt Sum1/1
  FixPt Constant/1 -> FixPt Relational Operator3/2, FixPt Data Type Duplicate/5, FixPt Sum1/2
  FixPt Sum1/1 -> FixPt Switch4/1, FixPt Data Type Duplicate/3

== system intertravamento/Additional Math & Discrete/Additional Math: Increment - Decrement/Decrement Time To Zero ==
  u : Inport
  FixPt Data Type Duplicate : DataTypeDuplicate  DisableCoverage=on  NumInputPorts=5
  FixPt Relational Operator3 : RelationalOperator  DisableCoverage=on  Operator=>  OutDataTypeStr=boolean  ZeroCross=off
  FixPt Sample Time Math : SampleTimeMath  DisableCoverage=on  TsampMathOp=Ts Only  OutDataTypeStr=Inherit: Inherit via back propagation
  FixPt Sum1 : Sum  DisableCoverage=on  Inputs=+-  OutDataTypeStr=Inherit: Inherit via back propagation  LockScale=on
  FixPt Switch4 : Switch  Criteria=u2 ~= 0  Threshold=1  OutDataTypeStr=Inherit: Inherit via back propagation  ZeroCross=off
  Ground1 : Ground  DisableCoverage=on
  y : Outport
  wires:
  FixPt Switch4/1 -> FixPt Data Type Duplicate/1, y/1
  Ground1/1 -> FixPt Data Type Duplicate/2, FixPt Switch4/3
  FixPt Relational Operator3/1 -> FixPt Switch4/2
  u/1 -> FixPt Relational Operator3/1, FixPt Data Type Duplicate/4, FixPt Sum1/1, FixPt Sample Time Math/1
  FixPt Sample Time Math/1 -> FixPt Relational Operator3/2, FixPt Data Type Duplicate/5, FixPt Sum1/2
  FixPt Sum1/1 -> FixPt Switch4/1, FixPt Data Type Duplicate/3

== system intertravamento/Additional Math & Discrete/Additional Math: Increment - Decrement/Increment Real World ==
  u : Inport
  FixPt Constant : Constant  DisableCoverage=on  OutDataTypeStr=Inherit: Inherit via back propagation
  FixPt Data Type Duplicate : DataTypeDuplicate  DisableCoverage=on  NumInputPorts=3
  FixPt Sum1 : Sum  OutDataTypeStr=Inherit: Inherit via back propagation  InputSameDT=on  LockScale=on
  y : Outport
  wires:
  u/1 -> FixPt Data Type Duplicate/2, FixPt Sum1/1
  FixPt Constant/1 -> FixPt Data Type Duplicate/3, FixPt Sum1/2
  FixPt Sum1/1 -> FixPt Data Type Duplicate/1, y/1

== system intertravamento/Additional Math & Discrete/Additional Math: Increment - Decrement/Increment Stored Integer ==
  u : Inport
  FixPt Constant : Constant  DisableCoverage=on  OutDataTypeStr=Inherit: Inherit via back propagation
  FixPt Data Type Duplicate : DataTypeDuplicate  DisableCoverage=on  NumInputPorts=3
  FixPt Data Type Propagation : simulink/Signal Attributes/Data Type Propagation  PropDataType=fixdt(1, 16)  IfRefDouble=double  IfRefSingle=single  IsSigned=IsSigned1  NumBitsBase=NumBits1  NumBitsMult=1  NumBitsAdd=0  NumBitsAllowFinal=1:128  PropScaling=2^-10  ValuesUsedBestPrec=[5 -7]  SlopeBase=Slope1  SlopeMult=0  SlopeAdd=1  BiasBase=Bias1  BiasMult=0  BiasAdd=0
  FixPt Gateway In : DataTypeConversion  DisableCoverage=on  ConvertRealWorld=Stored Integer (SI)
  FixPt Sum1 : Sum  OutDataTypeStr=Inherit: Inherit via back propagation  InputSameDT=on  LockScale=on
  y : Outport
  wires:
  FixPt Gateway In/1 -> FixPt Data Type Propagation/2, FixPt Data Type Propagation/1, FixPt Sum1/2, FixPt Data Type Duplicate/3
  FixPt Sum1/1 -> y/1, FixPt Data Type Duplicate/1
  FixPt Constant/1 -> FixPt Data Type Propagation/3, FixPt Gateway In/1
  u/1 -> FixPt Sum1/1, FixPt Data Type Duplicate/2

== system intertravamento/Model Verification/Check Input Resolution/fixed ==
  u : Inport
  resolution : Inport  Port=2
  fold : Logic  DisableCoverage=on  Operator=OR  Inputs=1
  relop : RelationalOperator  DisableCoverage=on  Operator===  InputSameDT=on
  out : Outport
  wires:
  u/1 -> relop/1
  resolution/1 -> relop/2
  relop/1 -> fold/1
  fold/1 -> out/1

== system intertravamento/Model Verification/Check Input Resolution/steps ==
  u : Inport
  resolution : Inport  Port=2
  relop : RelationalOperator  DisableCoverage=on  Operator=<=  InputSameDT=on
  rem : Math  DisableCoverage=on  Operator=mod  SaturateOnIntegerOverflow=on
  tol : Constant  DisableCoverage=on  Value=10e-3
  out : Outport
  wires:
  u/1 -> rem/1
  resolution/1 -> rem/2
  rem/1 -> relop/1
  tol/1 -> relop/2
  relop/1 -> out/1

== system intertravamento/Model-Wide Utilities/Block Support Table/EmptySubsystem ==

== system intertravamento/Model-Wide Utilities/DocBlock/EmptySubsystem ==

== system intertravamento/Model-Wide Utilities/Model Info/EmptySubsystem ==

== system intertravamento/Model-Wide Utilities/Timed-Based Linearization/Triggered Linearization ==
  Trigger : TriggerPort
  MATLAB S-Function : M-S-Function  DisableCoverage=on  FunctionName=sfunlin  Parameters=name_,SampleTime
